simulink library "PDBHandler"  (R2016b)
settings: Solver=VariableStepAuto  StartTime=0.0  StopTime=10.0  RelTol=1e-3
undefined symbols (not defined in the file or in its folder): PDBError
libraries: TimestampChecker x1
settings Model: Creator=Nathan  LastModifiedBy=MARCH

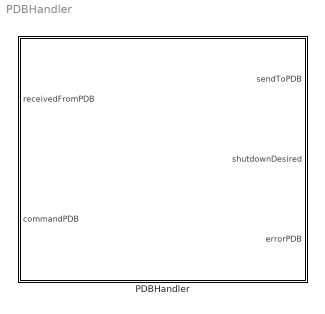
== system PDBHandler ==
  PDBHandler : Subsystem

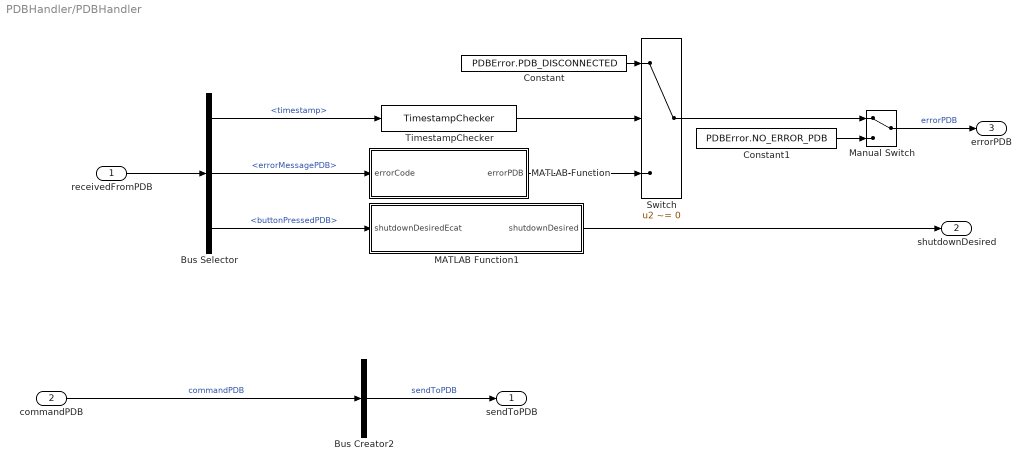
== system PDBHandler/PDBHandler ==
  receivedFromPDB : Inport  OutDataTypeStr=Bus: EtherCATReceivedFromPDB  BusOutputAsStruct=on
  commandPDB : Inport  Port=2
  Bus Creator2 : BusCreator  Inputs=1  OutDataTypeStr=Bus: EtherCATSendToPDB  NonVirtualBus=on
  Bus Selector : BusSelector  OutputSignals=timestamp,errorMessagePDB,buttonPressedPDB
  Constant : Constant  Value=PDBError.PDB_DISCONNECTED
  Constant1 : Constant  Value=PDBError.NO_ERROR_PDB
  MATLAB Function : MATLAB Function  TreatAsAtomicUnit=on
  MATLAB Function1 : MATLAB Function  TreatAsAtomicUnit=on
  Manual Switch : ManualSwitch
  Switch : Switch  Criteria=u2 ~= 0
  TimestampChecker : TimestampChecker/TimestampChecker
  sendToPDB : Outport  OutDataTypeStr=Bus: EtherCATSendToPDB
  shutdownDesired : Outport  Port=2
  errorPDB : Outport  Port=3
  wires:
  Manual Switch/1 -> errorPDB/1  "errorPDB"
  Bus Selector/3 -> MATLAB Function1/1(shutdownDesiredEcat)  "<buttonPressedPDB>"
  MATLAB Function1/1(shutdownDesired) -> shutdownDesired/1
  Constant1/1 -> Manual Switch/2
  Switch/1 -> Manual Switch/1
  Constant/1 -> Switch/1
  MATLAB Function/1(errorPDB) -> Switch/3
  TimestampChecker/1 -> Switch/2
  Bus Selector/1 -> TimestampChecker/1  "<timestamp>"
  Bus Selector/2 -> MATLAB Function/1(errorCode)  "<errorMessagePDB>"
  commandPDB/1 -> Bus Creator2/1  "commandPDB"
  receivedFromPDB/1 -> Bus Selector/1
  Bus Creator2/1 -> sendToPDB/1  "sendToPDB"

== matlab function PDBHandler/MATLAB Function1 ==
  data: shutdownDesiredEcat input; shutdownDesired output
function shutdownDesired = getShutdownDesired(shutdownDesiredEcat)
if shutdownDesiredEcat == 1
    shutdownDesired = 1;
else
    shutdownDesired = 0;
end

== matlab function PDBHandler/MATLAB Function ==
  data: errorCode input; errorPDB output
function errorPDB   = getPDBErrorFromErrorCode(errorCode)
% wrapper for getErrorFromErroCode
errorPDB = getPDBErrorFromErrorCode(errorCode);
end
